simulink model "model"  (R2016a)
settings: Solver=ode45  StartTime=0.0  StopTime=50  FixedStep=0.0001  RelTol=1e-4
values from neighbouring files (symbols this model uses):
  alpha = 0*pi/180    (= 0)    [Chassis_ss.m]    (also in ControllerDesign.m; RunHILsim.m; RunSimulation.m; plotFrame.m = 0.196349540849)
  b = 0    [Chassis_ss.m]    (also in ControllerDesign.m = 0.001; simulation.m = 0.005)
  c = 0    [Chassis_ss.m]    (also in ControllerDesign.m = 0.005; simulation.m = 0.005)
  g = 9.81    [Chassis_ss.m]    (also in ControllerDesign.m; RunHILsim.m; RunSimulation.m; simulation.m = 9.82)
  I = 0.007358820323616 - M*l^2    (= 0.00237702032362)    [Chassis_ss.m]    (also in ControllerDesign.m = 7.8125e-05; simulation.m = 7.8125e-05)
  J = ML_J + MR_J    (= -8.16854715147e-07)    [Chassis_ss.m]    (also in ControllerDesign.m = 3.22e-06; simulation.m = 3.22e-06)
  l = 95e-3    (= 0.095)    [Chassis_ss.m]    (also in ControllerDesign.m = 0.1; simulation.m = 0.5)
  M = 552e-3    (= 0.552)    [Chassis_ss.m]    (also in ControllerDesign.m = 0.8; simulation.m = 1)
  m = 452e-3    (= 0.452)    [Chassis_ss.m]    (also in ControllerDesign.m = 0.08; simulation.m = 0.5)
  r = (81.16*10^-3)/2    (= 0.04058)    [Chassis_ss.m]    (also in ControllerDesign.m = 0.045; atan2lookup.m = 1; plotFrame.m = 0.045; simulation.m = 0.045)
  theta0 = 10 * pi/180    (= 0.174532925199)    [ControllerDesign.m]    (also in RunHILsim.m = 0.436332312999; RunSimulation.m = 0.0872664625997; simulation.m = 0.0872664625997)
undefined symbols (not defined in the file or in its folder): K1, K2, p, p1
settings Model: Creator=masom  LastModifiedBy=Sam
settings SolverCC: ShapePreserveControl=EnableAll

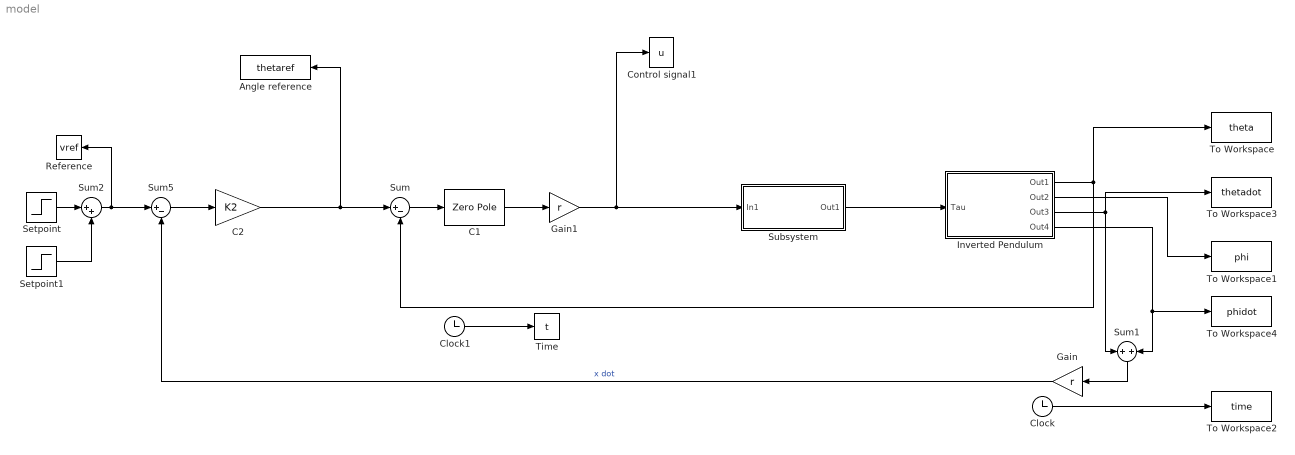
== system model ==
  Angle reference : ToWorkspace  VariableName=thetaref  SampleTime=-1
  C1 : ZeroPole  Zeros=[-p]  Poles=[-p1]  Gain=[K1]
  C2 : Gain  Gain=K2
  Clock : Clock
  Clock1 : Clock
  Control signal1 : ToWorkspace  VariableName=u  SampleTime=-1
  Gain : Gain  Gain=r
  Gain1 : Gain  Gain=r
  Inverted Pendulum : Subsystem
  Reference : ToWorkspace  VariableName=vref  SampleTime=-1
  Setpoint : Step  Time=10  After=0.5  SampleTime=0
  Setpoint1 : Step  Time=20  After=-0.5  SampleTime=0
  Subsystem : Subsystem
  Sum : Sum  Inputs=|+-
  Sum1 : Sum  Inputs=+|+
  Sum2 : Sum  Inputs=|++
  Sum5 : Sum  Inputs=|+-
  Time : ToWorkspace  VariableName=t  SampleTime=-1
  To Workspace : ToWorkspace  VariableName=theta  SampleTime=-1
  To Workspace1 : ToWorkspace  VariableName=phi  SampleTime=-1
  To Workspace2 : ToWorkspace  VariableName=time  SampleTime=-1
  To Workspace3 : ToWorkspace  VariableName=thetadot  SampleTime=-1
  To Workspace4 : ToWorkspace  VariableName=phidot  SampleTime=-1
  wires:
  Inverted Pendulum/2(Out2) -> To Workspace1/1
  Clock/1 -> To Workspace2/1
  Inverted Pendulum/3(Out3) -> To Workspace3/1, Sum1/1
  Inverted Pendulum/4(Out4) -> To Workspace4/1, Sum1/2
  Clock1/1 -> Time/1
  Sum/1 -> C1/1
  Gain/1 -> Sum5/2  "x dot"
  Inverted Pendulum/1(Out1) -> To Workspace/1, Sum/2
  Sum5/1 -> C2/1
  C2/1 -> Angle reference/1, Sum/1
  Setpoint/1 -> Sum2/1
  Setpoint1/1 -> Sum2/2
  Sum2/1 -> Sum5/1, Reference/1
  Sum1/1 -> Gain/1
  Gain1/1 -> Control signal1/1, Subsystem/1(In1)
  C1/1 -> Gain1/1
  Subsystem/1(Out1) -> Inverted Pendulum/1(Tau)

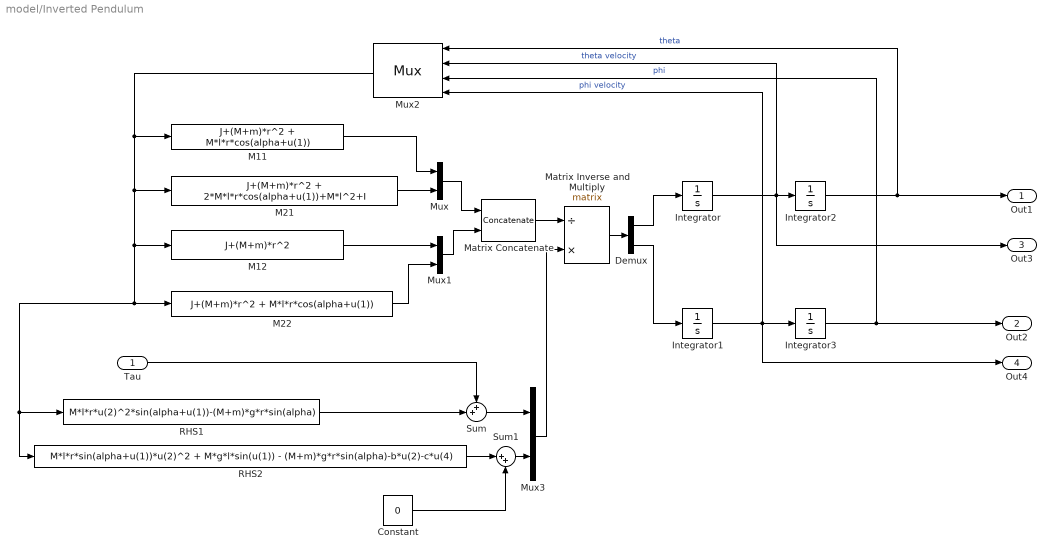
== system model/Inverted Pendulum ==
  Tau : Inport
  Constant : Constant  Value=0
  Demux : Demux  Outputs=2
  Integrator : Integrator  ContinuousStateAttributes='thetadot'
  Integrator1 : Integrator
  Integrator2 : Integrator  InitialCondition=theta0
  Integrator3 : Integrator
  "M11 " : Fcn  Expr=J+(M+m)*r^2 + M*l*r*cos(alpha+u(1))
  M12 : Fcn  Expr=J+(M+m)*r^2
  M21 : Fcn  Expr=J+(M+m)*r^2 + 2*M*l*r*cos(alpha+u(1))+M*l^2+I
  M22 : Fcn  Expr=J+(M+m)*r^2 + M*l*r*cos(alpha+u(1))
  Matrix Concatenate : Concatenate  Mode=Multidimensional array  ConcatenateDimension=2
  Matrix Inverse and Multiply : Product  Inputs=/*  Multiplication=Matrix(*)
  Mux : Mux  Inputs=2
  Mux1 : Mux  Inputs=2
  Mux2 : Mux
      settings: DisplayOption=signals
  Mux3 : Mux  Inputs=2
  RHS1 : Fcn  Expr=M*l*r*u(2)^2*sin(alpha+u(1))-(M+m)*g*r*sin(alpha)
  RHS2 : Fcn  Expr=M*l*r*sin(alpha+u(1))*u(2)^2 + M*g*l*sin(u(1)) - (M+m)*g*r*sin(alpha)-b*u(2)-c*u(4)
  Sum : Sum  Inputs=++|
  Sum1 : Sum  Inputs=|++
  Out1 : Outport
  Out2 : Outport  Port=2
  Out3 : Outport  Port=3
  Out4 : Outport  Port=4
  wires:
  M22/1 -> Mux1/2
  Integrator1/1 -> Out4/1, Mux2/4, Integrator3/1  "phi velocity"
  Demux/1 -> Integrator/1
  Mux/1 -> Matrix Concatenate/1
  Matrix Concatenate/1 -> Matrix Inverse and Multiply/1
  Demux/2 -> Integrator1/1
  Tau/1 -> Sum/1
  Mux1/1 -> Matrix Concatenate/2
  RHS1/1 -> Sum/2
  Matrix Inverse and Multiply/1 -> Demux/1
  Sum/1 -> Mux3/1
  Integrator/1 -> Out3/1, Mux2/2, Integrator2/1  "theta velocity"
  Integrator2/1 -> Out1/1, Mux2/1  "theta"
  Mux2/1 -> "M11 "/1, M12/1, M22/1, RHS1/1, RHS2/1, M21/1
  Mux3/1 -> Matrix Inverse and Multiply/2
  M21/1 -> Mux/2
  "M11 "/1 -> Mux/1
  Integrator3/1 -> Out2/1, Mux2/3  "phi"
  RHS2/1 -> Sum1/1
  Sum1/1 -> Mux3/2
  Constant/1 -> Sum1/2
  M12/1 -> Mux1/1

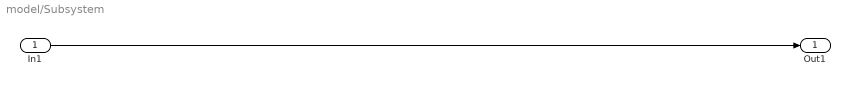
== system model/Subsystem ==
  In1 : Inport
  Out1 : Outport
  wires:
  In1/1 -> Out1/1
